simulink subsystem "resamplingtx"  (R2024b)
settings: Solver=VariableStepAuto  StartTime=0.0  StopTime=10.0  RelTol=1e-3
undefined symbols (not defined in the file or in its folder): a, b, c, c_resampling_0200, c_resampling_1071, c_resampling_2142, c_resampling_4473
libraries: hdlsllib x37
settings Model: Creator=usradmin  LastModifiedBy=jose.sanchez
settings RTWCC: GPUComputeCapability=3.5

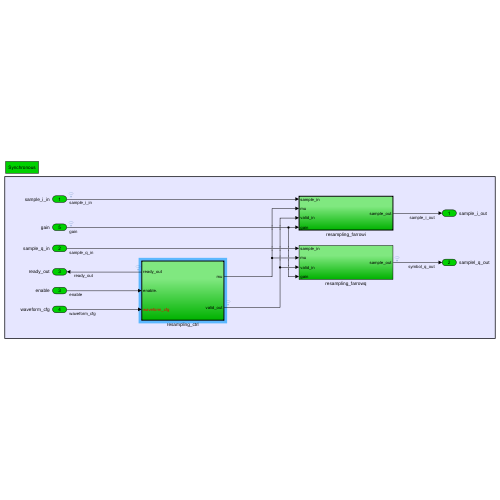
[thumbnail: Simulink's stored preview of the top-level diagram]
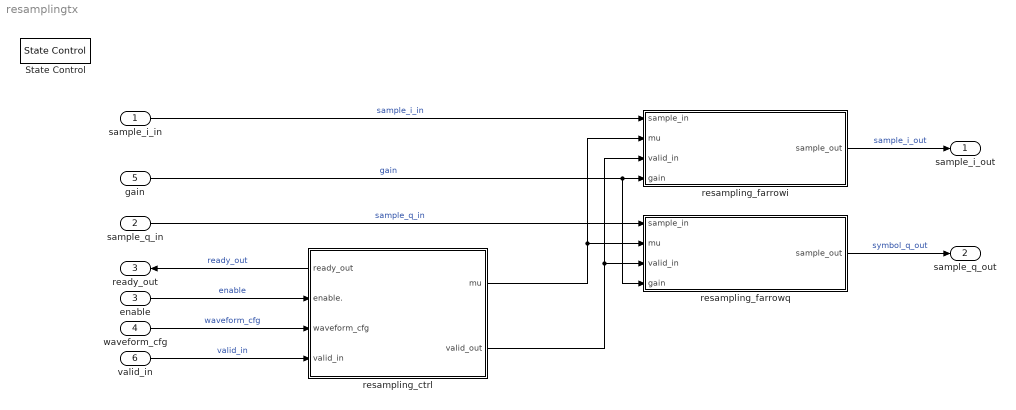
== system resamplingtx ==
  sample_i_in : Inport  OutDataTypeStr=fixdt(1,16,15)
  sample_q_in : Inport  Port=2  OutDataTypeStr=fixdt(1,16,15)
  enable : Inport  Port=3  OutDataTypeStr=boolean
  waveform_cfg : Inport  Port=4  OutDataTypeStr=fixdt(0,3,0)
  gain : Inport  Port=5  OutDataTypeStr=fixdt(1,17,14)
  valid_in : Inport  Port=6  OutDataTypeStr=boolean
  State Control : StateControl  StateControl=Synchronous
  resampling_ctrl : Subsystem
      settings: PortSchema="{\"entries\":[{\"content\":{\"sides\":[{\"content\":{\"connectorIds\":[\"Out3\",\"In1\",\"In2\",\"In3\"]},\"type\":\"ConnectorPlacement.EquallySpacedRectSide\",\"uuid\":\"3cd9d696-6190-459c-bb8b-8bb5d588c639\"},{\"content\":{\"connectorIds\":[\"Out1\",\"Out2\"],\"side\":\"RIGHT\"},\"type\":\"ConnectorPlacement.EquallySpacedRectSide\",\"uuid\":\"33a117ca-32f1-4181-9c0d-37c6fd5ec11a\"},{\"content\":{\"side\":\"TOP\"},\"type\":\"ConnectorPlacement.EquallySpacedRectSide\",\"uuid\":\"aa37b44e-ee4b-4e0b-b0bf-6dcd7e80fcbb\"}]},\"type\":\"ConnectorPlacement.EquallySpacedConnector\",\"uuid\":\"1cffff0a-15fe-4694-b57d-eb0cb56dd3c8\"}],\"packageUris\":[\"http://schema.mathworks.com/mf0/Connector/R2020b\"],\"version\":\"1.0\"}"
  resampling_farrowi : Subsystem
  resampling_farrowq : Subsystem  TreatAsAtomicUnit=on
  sample_i_out : Outport
  sample_q_out : Outport  Port=2
  ready_out : Outport  Port=3  OutDataTypeStr=boolean
  wires:
  sample_i_in/1 -> resampling_farrowi/1(sample_in)  "sample_i_in"
  resampling_farrowi/1(sample_out) -> sample_i_out/1  "sample_i_out"
  sample_q_in/1 -> resampling_farrowq/1(sample_in)  "sample_q_in"
  resampling_farrowq/1(sample_out) -> sample_q_out/1  "symbol_q_out"
  resampling_ctrl/2(valid_out) -> resampling_farrowi/3(valid_in), resampling_farrowq/3(valid_in)
  resampling_ctrl/3(ready_out) -> ready_out/1  "ready_out"
  enable/1 -> resampling_ctrl/1(enable.)  "enable"
  resampling_ctrl/1(mu) -> resampling_farrowi/2(mu), resampling_farrowq/2(mu)
  gain/1 -> resampling_farrowi/4(gain), resampling_farrowq/4(gain)  "gain"
  waveform_cfg/1 -> resampling_ctrl/2(waveform_cfg)  "waveform_cfg"
  valid_in/1 -> resampling_ctrl/3(valid_in)  "valid_in"

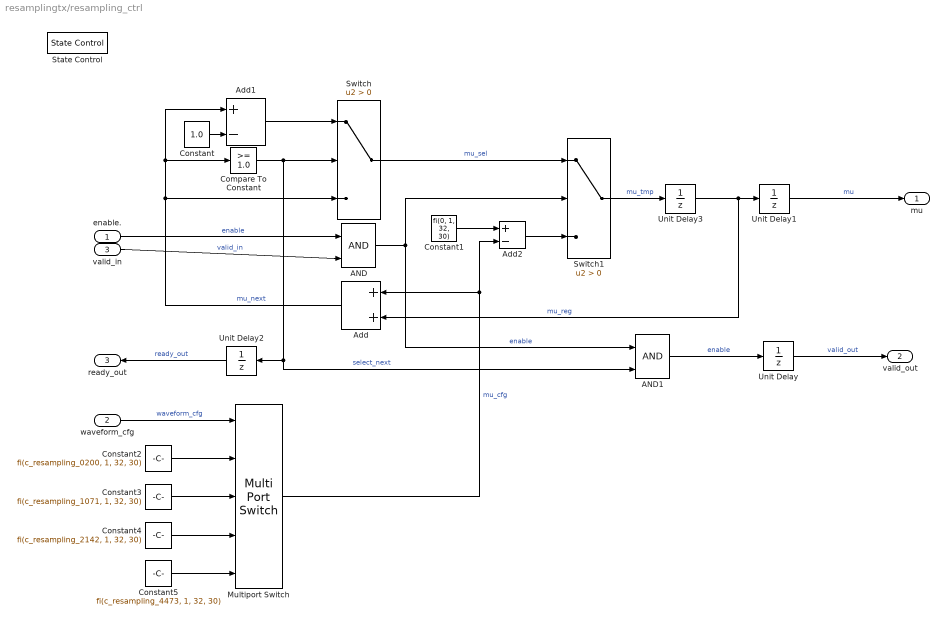
== system resamplingtx/resampling_ctrl ==
  enable. : Inport
  waveform_cfg : Inport  Port=2  OutDataTypeStr=fixdt(0,3,0)
  valid_in : Inport  Port=3
  AND : Logic  IconShape=distinctive  AllPortsSameDT=off  OutDataTypeStr=boolean
  AND1 : Logic  IconShape=distinctive  AllPortsSameDT=off  OutDataTypeStr=boolean
  Add : Sum
  Add1 : Sum  Inputs=+-
  Add2 : Sum  Inputs=+-
  Compare To Constant : hdlsllib/Logic and Bit Operations/Compare To Constant  relop=>=  const=1.0  OutDataTypeStr=boolean
  Constant : Constant  Value=1.0  OutDataTypeStr=fixdt(1,32,30)
  Constant1 : Constant  Value=fi(0, 1, 32, 30)
  Constant2 : Constant  Value=fi(c_resampling_0200, 1, 32, 30)
  Constant3 : Constant  Value=fi(c_resampling_1071, 1, 32, 30)
  Constant4 : Constant  Value=fi(c_resampling_2142, 1, 32, 30)
  Constant5 : Constant  Value=fi(c_resampling_4473, 1, 32, 30)
  Multiport Switch : MultiPortSwitch  Inputs=4  SaturateOnIntegerOverflow=off
  State Control : StateControl  StateControl=Synchronous
  Switch : Switch  Criteria=u2 > Threshold  SaturateOnIntegerOverflow=off  InputSameDT=off
  Switch1 : Switch  Criteria=u2 > Threshold  SaturateOnIntegerOverflow=off  InputSameDT=off
  Unit Delay{,1..3} (4 alike) : UnitDelay  SampleTime=-1  HasFrameUpgradeWarning=on
  mu : Outport  OutDataTypeStr=fixdt(1,32,30)
  valid_out : Outport  Port=2
  ready_out : Outport  Port=3
  wires:
  AND1/1 -> Unit Delay/1  "enable"
  valid_in/1 -> AND/2  "valid_in"
  enable./1 -> AND/1  "enable"
  Switch1/1 -> Unit Delay3/1  "mu_tmp"
  Add2/1 -> Switch1/3
  Constant1/1 -> Add2/1
  Switch/1 -> Switch1/1  "mu_sel"
  Unit Delay2/1 -> ready_out/1  "ready_out"
  Unit Delay1/1 -> mu/1  "mu"
  Unit Delay/1 -> valid_out/1  "valid_out"
  Compare To Constant/1 -> Switch/2, Unit Delay2/1, AND1/2  "select_next"
  Constant/1 -> Add1/2
  Unit Delay3/1 -> Unit Delay1/1, Add/2  "mu_reg"
  Add1/1 -> Switch/1
  Multiport Switch/1 -> Add2/2, Add/1  "mu_cfg"
  AND/1 -> Switch1/2, AND1/1  "enable"
  Add/1 -> Compare To Constant/1, Add1/1, Switch/3  "mu_next"
  waveform_cfg/1 -> Multiport Switch/1  "waveform_cfg"
  Constant2/1 -> Multiport Switch/2
  Constant3/1 -> Multiport Switch/3
  Constant4/1 -> Multiport Switch/4
  Constant5/1 -> Multiport Switch/5

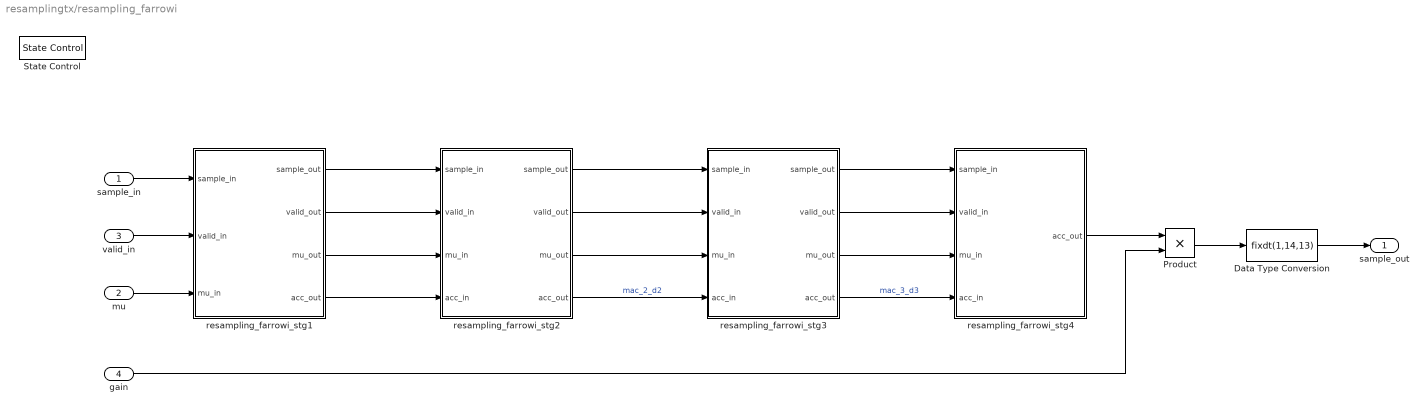
== system resamplingtx/resampling_farrowi ==
  sample_in : Inport
  mu : Inport  Port=2
  valid_in : Inport  Port=3
  gain : Inport  Port=4
  Data Type Conversion : DataTypeConversion  OutDataTypeStr=fixdt(1,14,13)  SaturateOnIntegerOverflow=off  RndMeth=Floor
  Product : Product
  State Control : StateControl  StateControl=Synchronous
  resampling_farrowi_stg1 : Subsystem
  resampling_farrowi_stg2 : Subsystem
  resampling_farrowi_stg3 : Subsystem
  resampling_farrowi_stg4 : Subsystem
  sample_out : Outport
  wires:
  mu/1 -> resampling_farrowi_stg1/3(mu_in)
  sample_in/1 -> resampling_farrowi_stg1/1(sample_in)
  valid_in/1 -> resampling_farrowi_stg1/2(valid_in)
  resampling_farrowi_stg1/1(sample_out) -> resampling_farrowi_stg2/1(sample_in)
  resampling_farrowi_stg1/2(valid_out) -> resampling_farrowi_stg2/2(valid_in)
  resampling_farrowi_stg1/3(mu_out) -> resampling_farrowi_stg2/3(mu_in)
  resampling_farrowi_stg1/4(acc_out) -> resampling_farrowi_stg2/4(acc_in)
  resampling_farrowi_stg2/1(sample_out) -> resampling_farrowi_stg3/1(sample_in)
  resampling_farrowi_stg2/2(valid_out) -> resampling_farrowi_stg3/2(valid_in)
  resampling_farrowi_stg2/3(mu_out) -> resampling_farrowi_stg3/3(mu_in)
  resampling_farrowi_stg2/4(acc_out) -> resampling_farrowi_stg3/4(acc_in)  "mac_2_d2"
  resampling_farrowi_stg3/1(sample_out) -> resampling_farrowi_stg4/1(sample_in)
  resampling_farrowi_stg3/2(valid_out) -> resampling_farrowi_stg4/2(valid_in)
  resampling_farrowi_stg3/3(mu_out) -> resampling_farrowi_stg4/3(mu_in)
  resampling_farrowi_stg3/4(acc_out) -> resampling_farrowi_stg4/4(acc_in)  "mac_3_d3"
  resampling_farrowi_stg4/1(acc_out) -> Product/1
  Product/1 -> Data Type Conversion/1
  gain/1 -> Product/2
  Data Type Conversion/1 -> sample_out/1

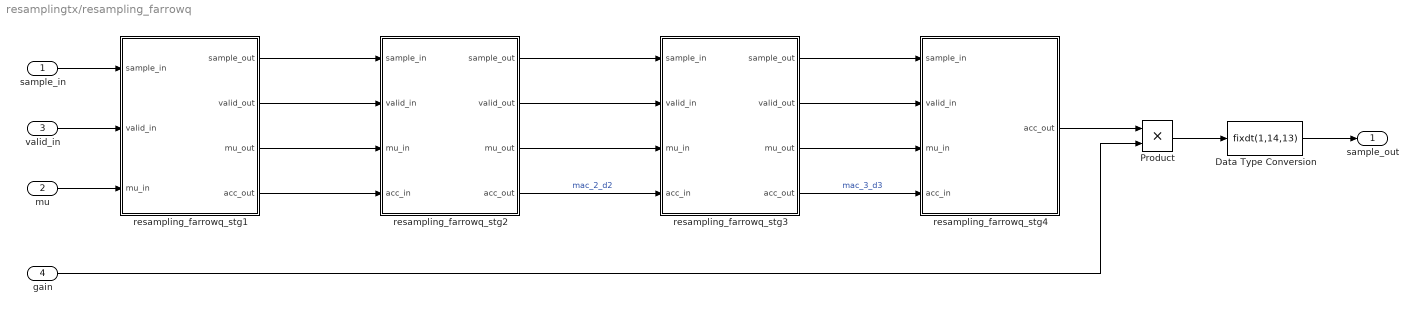
== system resamplingtx/resampling_farrowq ==
  sample_in : Inport
  mu : Inport  Port=2
  valid_in : Inport  Port=3
  gain : Inport  Port=4
  Data Type Conversion : DataTypeConversion  OutDataTypeStr=fixdt(1,14,13)  SaturateOnIntegerOverflow=off  RndMeth=Floor
  Product : Product
  resampling_farrowq_stg1 : Subsystem
  resampling_farrowq_stg2 : Subsystem
  resampling_farrowq_stg3 : Subsystem
  resampling_farrowq_stg4 : Subsystem
  sample_out : Outport
  wires:
  Data Type Conversion/1 -> sample_out/1
  gain/1 -> Product/2
  Product/1 -> Data Type Conversion/1
  resampling_farrowq_stg4/1(acc_out) -> Product/1
  resampling_farrowq_stg3/4(acc_out) -> resampling_farrowq_stg4/4(acc_in)  "mac_3_d3"
  resampling_farrowq_stg3/3(mu_out) -> resampling_farrowq_stg4/3(mu_in)
  resampling_farrowq_stg3/2(valid_out) -> resampling_farrowq_stg4/2(valid_in)
  resampling_farrowq_stg3/1(sample_out) -> resampling_farrowq_stg4/1(sample_in)
  resampling_farrowq_stg2/4(acc_out) -> resampling_farrowq_stg3/4(acc_in)  "mac_2_d2"
  resampling_farrowq_stg2/3(mu_out) -> resampling_farrowq_stg3/3(mu_in)
  resampling_farrowq_stg2/2(valid_out) -> resampling_farrowq_stg3/2(valid_in)
  resampling_farrowq_stg2/1(sample_out) -> resampling_farrowq_stg3/1(sample_in)
  resampling_farrowq_stg1/4(acc_out) -> resampling_farrowq_stg2/4(acc_in)
  resampling_farrowq_stg1/3(mu_out) -> resampling_farrowq_stg2/3(mu_in)
  resampling_farrowq_stg1/2(valid_out) -> resampling_farrowq_stg2/2(valid_in)
  resampling_farrowq_stg1/1(sample_out) -> resampling_farrowq_stg2/1(sample_in)
  valid_in/1 -> resampling_farrowq_stg1/2(valid_in)
  sample_in/1 -> resampling_farrowq_stg1/1(sample_in)
  mu/1 -> resampling_farrowq_stg1/3(mu_in)

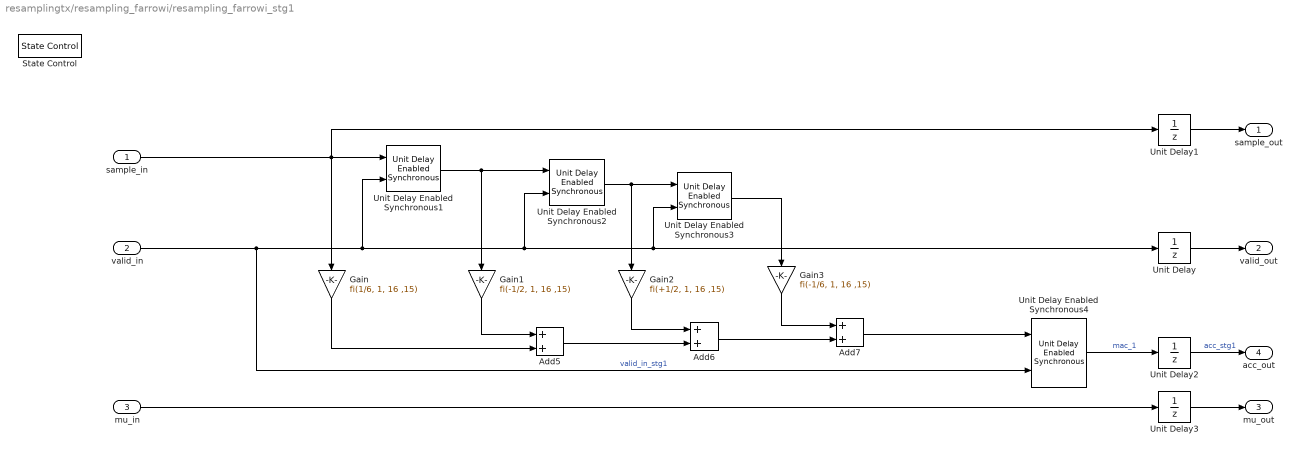
== system resamplingtx/resampling_farrowi/resampling_farrowi_stg1 ==
  sample_in : Inport  OutDataTypeStr=fixdt(1,16,15)
  valid_in : Inport  Port=2  OutDataTypeStr=boolean
  mu_in : Inport  Port=3
  Add5 : Sum
  Add6 : Sum
  Add7 : Sum
  Gain : Gain  Gain=fi(1/6, 1, 16 ,15)  OutDataTypeStr=fixdt(1,32,30)
  Gain1 : Gain  Gain=fi(-1/2, 1, 16 ,15)  OutDataTypeStr=fixdt(1,32,30)
  Gain2 : Gain  Gain=fi(+1/2, 1, 16 ,15)  OutDataTypeStr=fixdt(1,32,30)
  Gain3 : Gain  Gain=fi(-1/6, 1, 16 ,15)  OutDataTypeStr=fixdt(1,32,30)
  State Control : StateControl  StateControl=Synchronous
  Unit Delay{,1..3} (4 alike) : UnitDelay  SampleTime=-1  HasFrameUpgradeWarning=on
  Unit Delay Enabled Synchronous{1..4} (4 alike) : hdlsllib/Discrete/Unit Delay Enabled Synchronous  InitialCondition=0.0  SampleTime=-1
  sample_out : Outport  OutDataTypeStr=fixdt(1,16,15)
  valid_out : Outport  Port=2  OutDataTypeStr=boolean
  mu_out : Outport  Port=3
  acc_out : Outport  Port=4
  wires:
  Unit Delay Enabled Synchronous4/1 -> Unit Delay2/1  "mac_1"
  Add7/1 -> Unit Delay Enabled Synchronous4/1
  Unit Delay Enabled Synchronous3/1 -> Gain3/1
  valid_in/1 -> Unit Delay Enabled Synchronous4/2, Unit Delay Enabled Synchronous1/2, Unit Delay Enabled Synchronous2/2, Unit Delay Enabled Synchronous3/2, Unit Delay/1  "valid_in_stg1"
  sample_in/1 -> Gain/1, Unit Delay Enabled Synchronous1/1, Unit Delay1/1
  Add5/1 -> Add6/2
  Gain3/1 -> Add7/1
  Unit Delay Enabled Synchronous2/1 -> Gain2/1, Unit Delay Enabled Synchronous3/1
  Gain1/1 -> Add5/1
  Add6/1 -> Add7/2
  Gain/1 -> Add5/2
  Gain2/1 -> Add6/1
  Unit Delay Enabled Synchronous1/1 -> Gain1/1, Unit Delay Enabled Synchronous2/1
  mu_in/1 -> Unit Delay3/1
  Unit Delay1/1 -> sample_out/1
  Unit Delay/1 -> valid_out/1
  Unit Delay2/1 -> acc_out/1  "acc_stg1"
  Unit Delay3/1 -> mu_out/1

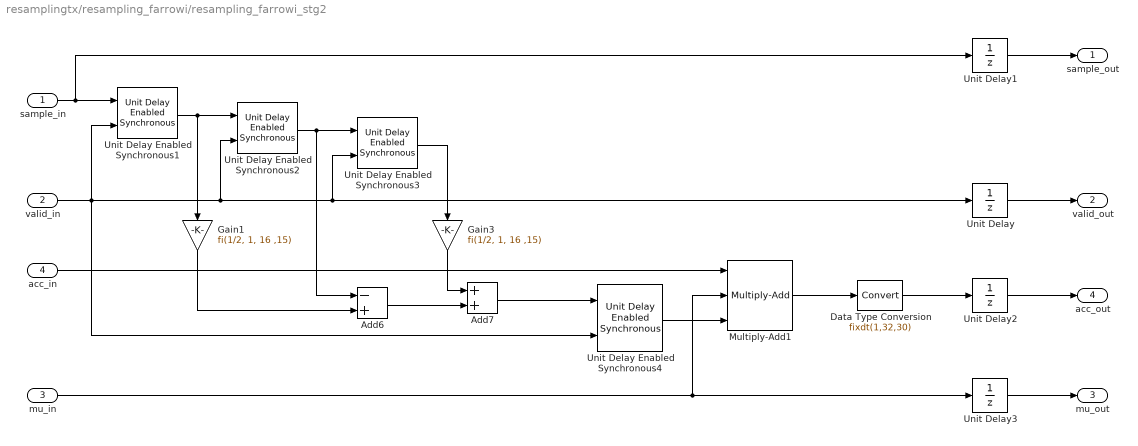
== system resamplingtx/resampling_farrowi/resampling_farrowi_stg2 ==
  sample_in : Inport  OutDataTypeStr=fixdt(1,16,15)
  valid_in : Inport  Port=2  OutDataTypeStr=boolean
  mu_in : Inport  Port=3
  acc_in : Inport  Port=4
  Add6 : Sum  Inputs=-+
  Add7 : Sum
  Data Type Conversion : DataTypeConversion  OutDataTypeStr=fixdt(1,32,30)  SaturateOnIntegerOverflow=off  RndMeth=Floor
  Gain1 : Gain  Gain=fi(1/2, 1, 16 ,15)  OutDataTypeStr=fixdt(1,32,30)
  Gain3 : Gain  Gain=fi(1/2, 1, 16 ,15)  OutDataTypeStr=fixdt(1,32,30)
  Multiply-Add1 : hdlsllib/HDL Operations/Multiply-Add  Function=c+(a.*b)  datatype=Inherit: Inherit via internal rule  DoSatur=off  FMA=off
  Unit Delay{,1..3} (4 alike) : UnitDelay  SampleTime=-1  HasFrameUpgradeWarning=on
  Unit Delay Enabled Synchronous{1..4} (4 alike) : hdlsllib/Discrete/Unit Delay Enabled Synchronous  InitialCondition=0.0  SampleTime=-1
  sample_out : Outport  OutDataTypeStr=fixdt(1,16,15)
  valid_out : Outport  Port=2  OutDataTypeStr=boolean
  mu_out : Outport  Port=3
  acc_out : Outport  Port=4
  wires:
  Unit Delay Enabled Synchronous4/1 -> Multiply-Add1/3
  Add7/1 -> Unit Delay Enabled Synchronous4/1
  Data Type Conversion/1 -> Unit Delay2/1
  Unit Delay3/1 -> mu_out/1
  Unit Delay2/1 -> acc_out/1
  Unit Delay/1 -> valid_out/1
  Unit Delay1/1 -> sample_out/1
  mu_in/1 -> Unit Delay3/1, Multiply-Add1/2
  Multiply-Add1/1 -> Data Type Conversion/1
  acc_in/1 -> Multiply-Add1/1
  Unit Delay Enabled Synchronous1/1 -> Gain1/1, Unit Delay Enabled Synchronous2/1
  Unit Delay Enabled Synchronous2/1 -> Add6/1, Unit Delay Enabled Synchronous3/1
  Add6/1 -> Add7/2
  Gain1/1 -> Add6/2
  Gain3/1 -> Add7/1
  sample_in/1 -> Unit Delay Enabled Synchronous1/1, Unit Delay1/1
  valid_in/1 -> Unit Delay Enabled Synchronous1/2, Unit Delay Enabled Synchronous4/2, Unit Delay Enabled Synchronous2/2, Unit Delay Enabled Synchronous3/2, Unit Delay/1
  Unit Delay Enabled Synchronous3/1 -> Gain3/1

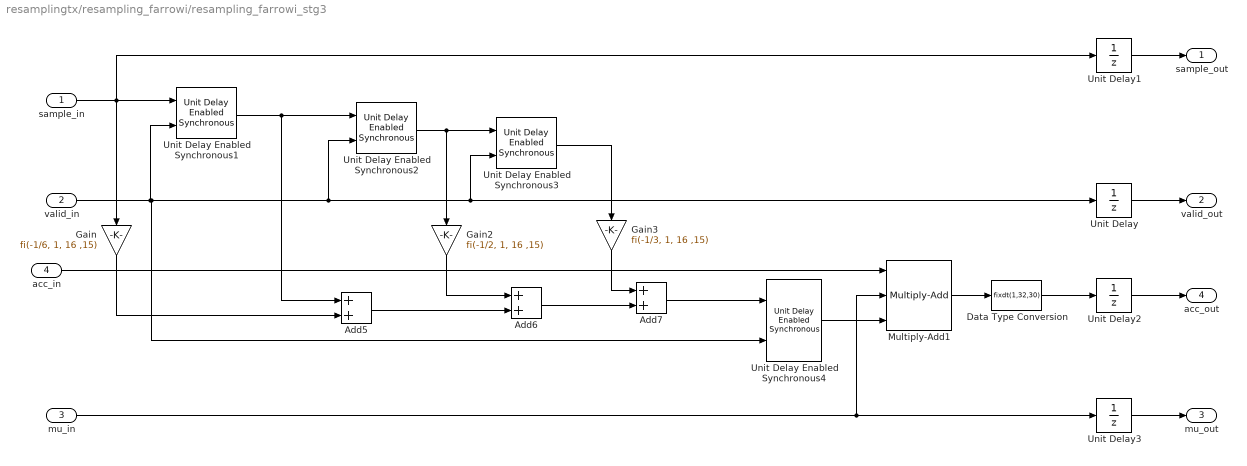
== system resamplingtx/resampling_farrowi/resampling_farrowi_stg3 ==
  sample_in : Inport  OutDataTypeStr=fixdt(1,16,15)
  valid_in : Inport  Port=2  OutDataTypeStr=boolean
  mu_in : Inport  Port=3
  acc_in : Inport  Port=4
  Add5 : Sum
  Add6 : Sum
  Add7 : Sum
  Data Type Conversion : DataTypeConversion  OutDataTypeStr=fixdt(1,32,30)  SaturateOnIntegerOverflow=off  RndMeth=Floor
  Gain : Gain  Gain=fi(-1/6, 1, 16 ,15)  OutDataTypeStr=fixdt(1,32,30)
  Gain2 : Gain  Gain=fi(-1/2, 1, 16 ,15)  OutDataTypeStr=fixdt(1,32,30)
  Gain3 : Gain  Gain=fi(-1/3, 1, 16 ,15)  OutDataTypeStr=fixdt(1,32,30)
  Multiply-Add1 : hdlsllib/HDL Operations/Multiply-Add  Function=c+(a.*b)  datatype=Inherit: Inherit via internal rule  DoSatur=off  FMA=off
  Unit Delay{,1..3} (4 alike) : UnitDelay  SampleTime=-1  HasFrameUpgradeWarning=on
  Unit Delay Enabled Synchronous{1..4} (4 alike) : hdlsllib/Discrete/Unit Delay Enabled Synchronous  InitialCondition=0.0  SampleTime=-1
  sample_out : Outport  OutDataTypeStr=fixdt(1,16,15)
  valid_out : Outport  Port=2  OutDataTypeStr=boolean
  mu_out : Outport  Port=3
  acc_out : Outport  Port=4
  wires:
  Unit Delay Enabled Synchronous4/1 -> Multiply-Add1/3
  Add7/1 -> Unit Delay Enabled Synchronous4/1
  Data Type Conversion/1 -> Unit Delay2/1
  Unit Delay Enabled Synchronous3/1 -> Gain3/1
  valid_in/1 -> Unit Delay Enabled Synchronous1/2, Unit Delay Enabled Synchronous4/2, Unit Delay Enabled Synchronous2/2, Unit Delay/1, Unit Delay Enabled Synchronous3/2
  sample_in/1 -> Gain/1, Unit Delay Enabled Synchronous1/1, Unit Delay1/1
  Add5/1 -> Add6/2
  Gain3/1 -> Add7/1
  Unit Delay Enabled Synchronous2/1 -> Gain2/1, Unit Delay Enabled Synchronous3/1
  Unit Delay Enabled Synchronous1/1 -> Add5/1, Unit Delay Enabled Synchronous2/1
  Add6/1 -> Add7/2
  Gain/1 -> Add5/2
  Gain2/1 -> Add6/1
  acc_in/1 -> Multiply-Add1/1
  Multiply-Add1/1 -> Data Type Conversion/1
  mu_in/1 -> Multiply-Add1/2, Unit Delay3/1
  Unit Delay1/1 -> sample_out/1
  Unit Delay/1 -> valid_out/1
  Unit Delay2/1 -> acc_out/1
  Unit Delay3/1 -> mu_out/1

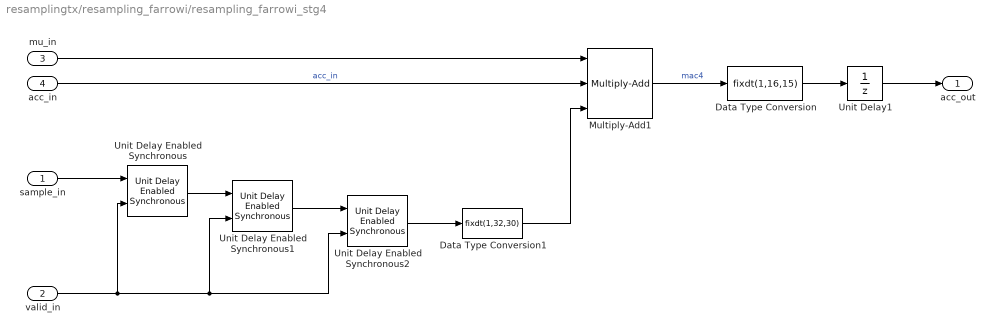
== system resamplingtx/resampling_farrowi/resampling_farrowi_stg4 ==
  sample_in : Inport  OutDataTypeStr=fixdt(1,16,15)
  valid_in : Inport  Port=2  OutDataTypeStr=boolean
  mu_in : Inport  Port=3
  acc_in : Inport  Port=4
  Data Type Conversion : DataTypeConversion  OutDataTypeStr=fixdt(1,16,15)  SaturateOnIntegerOverflow=off  RndMeth=Floor
  Data Type Conversion1 : DataTypeConversion  OutDataTypeStr=fixdt(1,32,30)  SaturateOnIntegerOverflow=off  RndMeth=Floor
  Multiply-Add1 : hdlsllib/HDL Operations/Multiply-Add  Function=c+(a.*b)  datatype=Inherit: Inherit via internal rule  DoSatur=off  FMA=off
  Unit Delay Enabled Synchronous : hdlsllib/Discrete/Unit Delay Enabled Synchronous  InitialCondition=0.0  SampleTime=-1
  Unit Delay Enabled Synchronous1 : hdlsllib/Discrete/Unit Delay Enabled Synchronous  InitialCondition=0.0  SampleTime=-1
  Unit Delay Enabled Synchronous2 : hdlsllib/Discrete/Unit Delay Enabled Synchronous  InitialCondition=0.0  SampleTime=-1
  Unit Delay1 : UnitDelay  SampleTime=-1  HasFrameUpgradeWarning=on
  acc_out : Outport
  wires:
  Data Type Conversion1/1 -> Multiply-Add1/3
  Unit Delay Enabled Synchronous2/1 -> Data Type Conversion1/1
  Unit Delay Enabled Synchronous1/1 -> Unit Delay Enabled Synchronous2/1
  Multiply-Add1/1 -> Data Type Conversion/1  "mac4"
  Unit Delay1/1 -> acc_out/1
  mu_in/1 -> Multiply-Add1/1
  acc_in/1 -> Multiply-Add1/2  "acc_in"
  Unit Delay Enabled Synchronous/1 -> Unit Delay Enabled Synchronous1/1
  valid_in/1 -> Unit Delay Enabled Synchronous2/2, Unit Delay Enabled Synchronous1/2, Unit Delay Enabled Synchronous/2
  sample_in/1 -> Unit Delay Enabled Synchronous/1
  Data Type Conversion/1 -> Unit Delay1/1

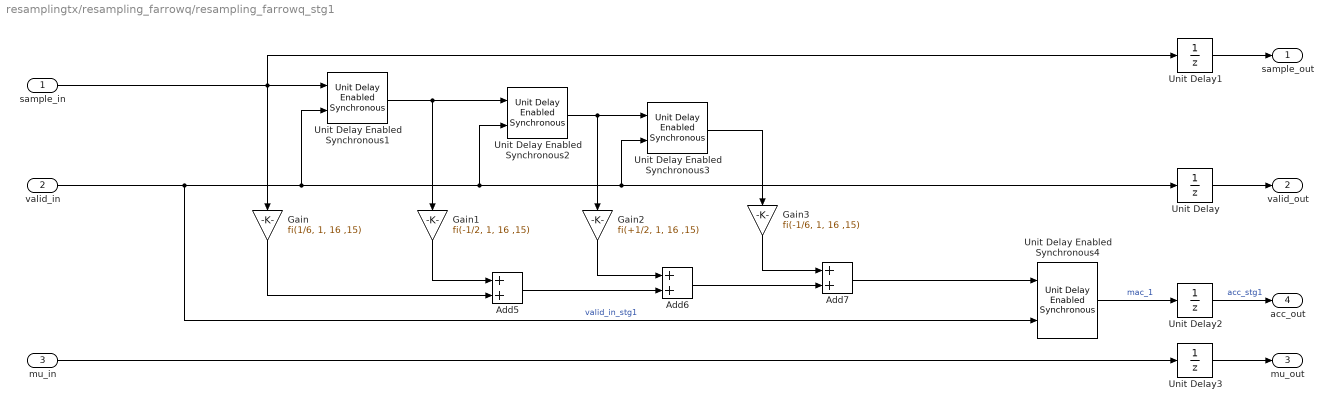
== system resamplingtx/resampling_farrowq/resampling_farrowq_stg1 ==
  sample_in : Inport  OutDataTypeStr=fixdt(1,16,15)
  valid_in : Inport  Port=2  OutDataTypeStr=boolean
  mu_in : Inport  Port=3
  Add5 : Sum
  Add6 : Sum
  Add7 : Sum
  Gain : Gain  Gain=fi(1/6, 1, 16 ,15)  OutDataTypeStr=fixdt(1,32,30)
  Gain1 : Gain  Gain=fi(-1/2, 1, 16 ,15)  OutDataTypeStr=fixdt(1,32,30)
  Gain2 : Gain  Gain=fi(+1/2, 1, 16 ,15)  OutDataTypeStr=fixdt(1,32,30)
  Gain3 : Gain  Gain=fi(-1/6, 1, 16 ,15)  OutDataTypeStr=fixdt(1,32,30)
  Unit Delay{,1..3} (4 alike) : UnitDelay  SampleTime=-1  HasFrameUpgradeWarning=on
  Unit Delay Enabled Synchronous{1..4} (4 alike) : hdlsllib/Discrete/Unit Delay Enabled Synchronous  InitialCondition=0.0  SampleTime=-1
  sample_out : Outport  OutDataTypeStr=fixdt(1,16,15)
  valid_out : Outport  Port=2  OutDataTypeStr=boolean
  mu_out : Outport  Port=3
  acc_out : Outport  Port=4
  wires:
  Unit Delay3/1 -> mu_out/1
  Unit Delay2/1 -> acc_out/1  "acc_stg1"
  Unit Delay/1 -> valid_out/1
  Unit Delay1/1 -> sample_out/1
  mu_in/1 -> Unit Delay3/1
  Unit Delay Enabled Synchronous1/1 -> Unit Delay Enabled Synchronous2/1, Gain1/1
  Gain2/1 -> Add6/1
  Gain/1 -> Add5/2
  Add6/1 -> Add7/2
  Gain1/1 -> Add5/1
  Unit Delay Enabled Synchronous2/1 -> Unit Delay Enabled Synchronous3/1, Gain2/1
  Gain3/1 -> Add7/1
  Add5/1 -> Add6/2
  sample_in/1 -> Unit Delay1/1, Unit Delay Enabled Synchronous1/1, Gain/1
  valid_in/1 -> Unit Delay/1, Unit Delay Enabled Synchronous3/2, Unit Delay Enabled Synchronous2/2, Unit Delay Enabled Synchronous1/2, Unit Delay Enabled Synchronous4/2  "valid_in_stg1"
  Unit Delay Enabled Synchronous3/1 -> Gain3/1
  Add7/1 -> Unit Delay Enabled Synchronous4/1
  Unit Delay Enabled Synchronous4/1 -> Unit Delay2/1  "mac_1"

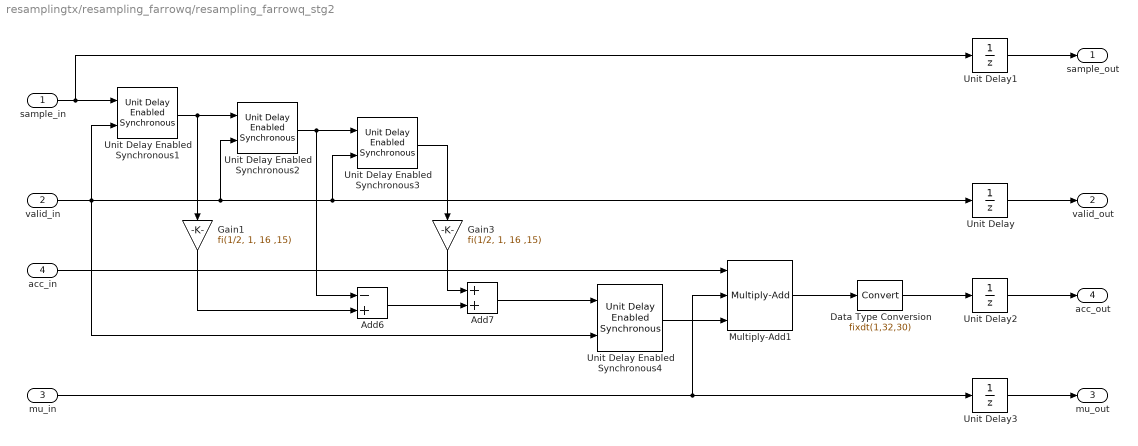
== system resamplingtx/resampling_farrowq/resampling_farrowq_stg2 ==
  sample_in : Inport  OutDataTypeStr=fixdt(1,16,15)
  valid_in : Inport  Port=2  OutDataTypeStr=boolean
  mu_in : Inport  Port=3
  acc_in : Inport  Port=4
  Add6 : Sum  Inputs=-+
  Add7 : Sum
  Data Type Conversion : DataTypeConversion  OutDataTypeStr=fixdt(1,32,30)  SaturateOnIntegerOverflow=off  RndMeth=Floor
  Gain1 : Gain  Gain=fi(1/2, 1, 16 ,15)  OutDataTypeStr=fixdt(1,32,30)
  Gain3 : Gain  Gain=fi(1/2, 1, 16 ,15)  OutDataTypeStr=fixdt(1,32,30)
  Multiply-Add1 : hdlsllib/HDL Operations/Multiply-Add  Function=c+(a.*b)  datatype=Inherit: Inherit via internal rule  DoSatur=off  FMA=off
  Unit Delay{,1..3} (4 alike) : UnitDelay  SampleTime=-1  HasFrameUpgradeWarning=on
  Unit Delay Enabled Synchronous{1..4} (4 alike) : hdlsllib/Discrete/Unit Delay Enabled Synchronous  InitialCondition=0.0  SampleTime=-1
  sample_out : Outport  OutDataTypeStr=fixdt(1,16,15)
  valid_out : Outport  Port=2  OutDataTypeStr=boolean
  mu_out : Outport  Port=3
  acc_out : Outport  Port=4
  wires:
  Unit Delay Enabled Synchronous3/1 -> Gain3/1
  valid_in/1 -> Unit Delay/1, Unit Delay Enabled Synchronous3/2, Unit Delay Enabled Synchronous2/2, Unit Delay Enabled Synchronous4/2, Unit Delay Enabled Synchronous1/2
  sample_in/1 -> Unit Delay1/1, Unit Delay Enabled Synchronous1/1
  Gain3/1 -> Add7/1
  Gain1/1 -> Add6/2
  Add6/1 -> Add7/2
  Unit Delay Enabled Synchronous2/1 -> Unit Delay Enabled Synchronous3/1, Add6/1
  Unit Delay Enabled Synchronous1/1 -> Unit Delay Enabled Synchronous2/1, Gain1/1
  acc_in/1 -> Multiply-Add1/1
  Multiply-Add1/1 -> Data Type Conversion/1
  mu_in/1 -> Multiply-Add1/2, Unit Delay3/1
  Unit Delay1/1 -> sample_out/1
  Unit Delay/1 -> valid_out/1
  Unit Delay2/1 -> acc_out/1
  Unit Delay3/1 -> mu_out/1
  Data Type Conversion/1 -> Unit Delay2/1
  Add7/1 -> Unit Delay Enabled Synchronous4/1
  Unit Delay Enabled Synchronous4/1 -> Multiply-Add1/3

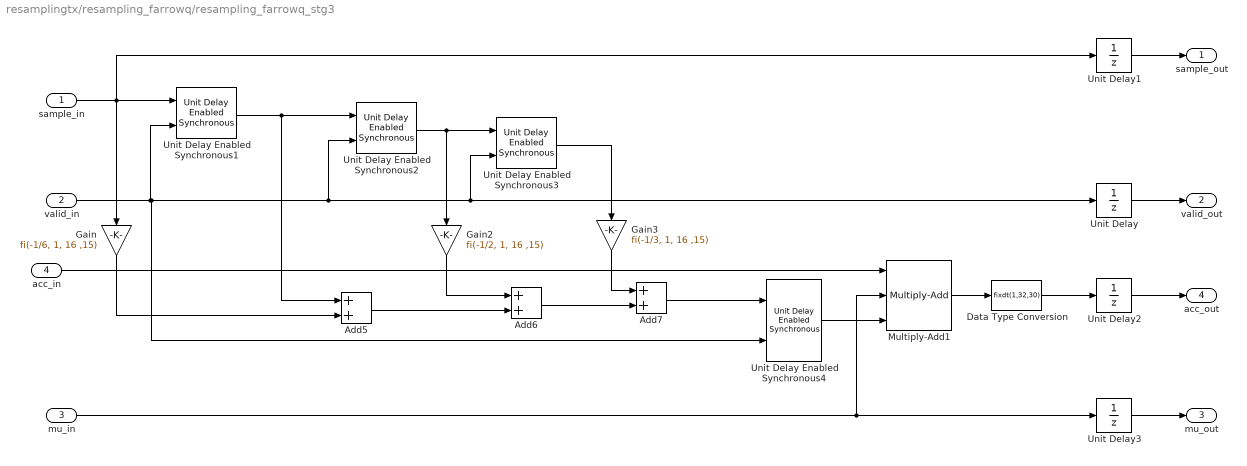
== system resamplingtx/resampling_farrowq/resampling_farrowq_stg3 ==
  sample_in : Inport  OutDataTypeStr=fixdt(1,16,15)
  valid_in : Inport  Port=2  OutDataTypeStr=boolean
  mu_in : Inport  Port=3
  acc_in : Inport  Port=4
  Add5 : Sum
  Add6 : Sum
  Add7 : Sum
  Data Type Conversion : DataTypeConversion  OutDataTypeStr=fixdt(1,32,30)  SaturateOnIntegerOverflow=off  RndMeth=Floor
  Gain : Gain  Gain=fi(-1/6, 1, 16 ,15)  OutDataTypeStr=fixdt(1,32,30)
  Gain2 : Gain  Gain=fi(-1/2, 1, 16 ,15)  OutDataTypeStr=fixdt(1,32,30)
  Gain3 : Gain  Gain=fi(-1/3, 1, 16 ,15)  OutDataTypeStr=fixdt(1,32,30)
  Multiply-Add1 : hdlsllib/HDL Operations/Multiply-Add  Function=c+(a.*b)  datatype=Inherit: Inherit via internal rule  DoSatur=off  FMA=off
  Unit Delay{,1..3} (4 alike) : UnitDelay  SampleTime=-1  HasFrameUpgradeWarning=on
  Unit Delay Enabled Synchronous{1..4} (4 alike) : hdlsllib/Discrete/Unit Delay Enabled Synchronous  InitialCondition=0.0  SampleTime=-1
  sample_out : Outport  OutDataTypeStr=fixdt(1,16,15)
  valid_out : Outport  Port=2  OutDataTypeStr=boolean
  mu_out : Outport  Port=3
  acc_out : Outport  Port=4
  wires:
  Unit Delay3/1 -> mu_out/1
  Unit Delay2/1 -> acc_out/1
  Unit Delay/1 -> valid_out/1
  Unit Delay1/1 -> sample_out/1
  mu_in/1 -> Unit Delay3/1, Multiply-Add1/2
  Multiply-Add1/1 -> Data Type Conversion/1
  acc_in/1 -> Multiply-Add1/1
  Gain2/1 -> Add6/1
  Gain/1 -> Add5/2
  Add6/1 -> Add7/2
  Unit Delay Enabled Synchronous1/1 -> Unit Delay Enabled Synchronous2/1, Add5/1
  Unit Delay Enabled Synchronous2/1 -> Unit Delay Enabled Synchronous3/1, Gain2/1
  Gain3/1 -> Add7/1
  Add5/1 -> Add6/2
  sample_in/1 -> Unit Delay1/1, Unit Delay Enabled Synchronous1/1, Gain/1
  valid_in/1 -> Unit Delay Enabled Synchronous3/2, Unit Delay/1, Unit Delay Enabled Synchronous2/2, Unit Delay Enabled Synchronous4/2, Unit Delay Enabled Synchronous1/2
  Unit Delay Enabled Synchronous3/1 -> Gain3/1
  Data Type Conversion/1 -> Unit Delay2/1
  Add7/1 -> Unit Delay Enabled Synchronous4/1
  Unit Delay Enabled Synchronous4/1 -> Multiply-Add1/3

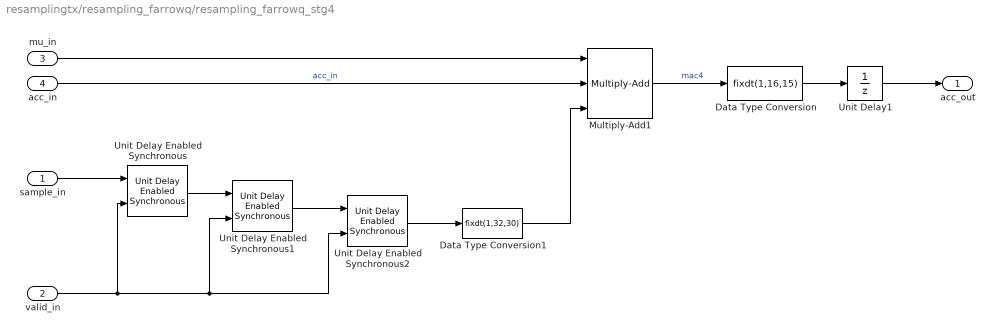
== system resamplingtx/resampling_farrowq/resampling_farrowq_stg4 ==
  sample_in : Inport  OutDataTypeStr=fixdt(1,16,15)
  valid_in : Inport  Port=2  OutDataTypeStr=boolean
  mu_in : Inport  Port=3
  acc_in : Inport  Port=4
  Data Type Conversion : DataTypeConversion  OutDataTypeStr=fixdt(1,16,15)  SaturateOnIntegerOverflow=off  RndMeth=Floor
  Data Type Conversion1 : DataTypeConversion  OutDataTypeStr=fixdt(1,32,30)  SaturateOnIntegerOverflow=off  RndMeth=Floor
  Multiply-Add1 : hdlsllib/HDL Operations/Multiply-Add  Function=c+(a.*b)  datatype=Inherit: Inherit via internal rule  DoSatur=off  FMA=off
  Unit Delay Enabled Synchronous : hdlsllib/Discrete/Unit Delay Enabled Synchronous  InitialCondition=0.0  SampleTime=-1
  Unit Delay Enabled Synchronous1 : hdlsllib/Discrete/Unit Delay Enabled Synchronous  InitialCondition=0.0  SampleTime=-1
  Unit Delay Enabled Synchronous2 : hdlsllib/Discrete/Unit Delay Enabled Synchronous  InitialCondition=0.0  SampleTime=-1
  Unit Delay1 : UnitDelay  SampleTime=-1  HasFrameUpgradeWarning=on
  acc_out : Outport
  wires:
  Data Type Conversion/1 -> Unit Delay1/1
  sample_in/1 -> Unit Delay Enabled Synchronous/1
  valid_in/1 -> Unit Delay Enabled Synchronous/2, Unit Delay Enabled Synchronous1/2, Unit Delay Enabled Synchronous2/2
  Unit Delay Enabled Synchronous/1 -> Unit Delay Enabled Synchronous1/1
  acc_in/1 -> Multiply-Add1/2  "acc_in"
  mu_in/1 -> Multiply-Add1/1
  Unit Delay1/1 -> acc_out/1
  Multiply-Add1/1 -> Data Type Conversion/1  "mac4"
  Unit Delay Enabled Synchronous1/1 -> Unit Delay Enabled Synchronous2/1
  Unit Delay Enabled Synchronous2/1 -> Data Type Conversion1/1
  Data Type Conversion1/1 -> Multiply-Add1/3
